simulink subsystem "motor_velocity_loop_model_v2"  (R2023b)
settings: Solver=VariableStepAuto  StartTime=0.0  StopTime=10.0  RelTol=1e-3
values from neighbouring files (symbols this model uses):
  omega_in_bar_dt_max = 628.318530718    [mdl_parameters_int.mat]
  omega_in_bar_dt_min = -1047.1975512    [mdl_parameters_int.mat]
  omega_in_max = 397.935069455    [mdl_parameters_int.mat]
  omega_in_min = 0    [mdl_parameters_int.mat]
  tau_s = 0.0005    [mdl_parameters_int.mat]
undefined symbols (not defined in the file or in its folder): T_omega_in
libraries: cstblocks x2
settings Model: Creator=Previ  LastModifiedBy=Previ

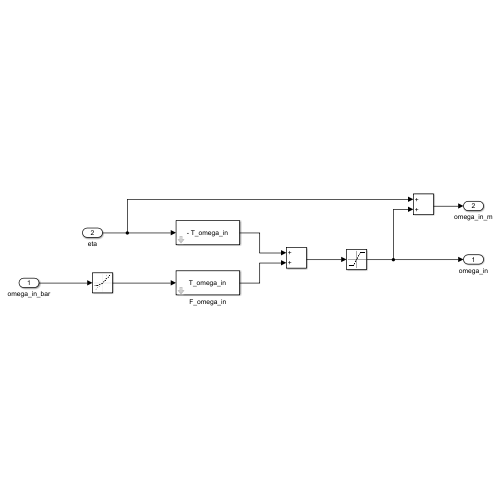
[thumbnail: Simulink's stored preview of the top-level diagram]
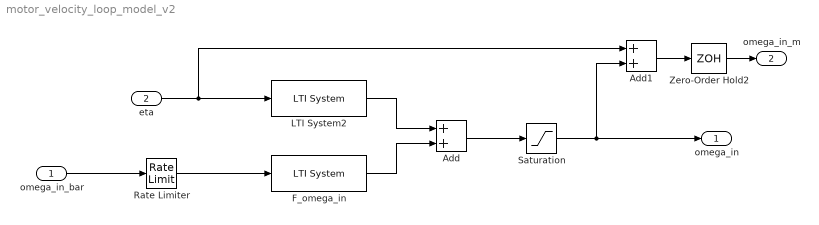
== system motor_velocity_loop_model_v2 ==
  omega_in_bar : Inport  PortDimensions=[1, 1]
  eta : Inport  Port=2  PortDimensions=[1, 1]
  Add : Sum
  Add1 : Sum
  F_omega_in : cstblocks/LTI System  sys=T_omega_in  IC=[]  PadeOrder=0
  LTI System2 : cstblocks/LTI System  sys=- T_omega_in  IC=[]  PadeOrder=0
  Rate Limiter : RateLimiter  RisingSlewLimit=omega_in_bar_dt_max  FallingSlewLimit=omega_in_bar_dt_min  SampleTimeMode=inherited
  Saturation : Saturate  UpperLimit=omega_in_max  LowerLimit=omega_in_min
  Zero-Order Hold2 : ZeroOrderHold  SampleTime=tau_s
  omega_in : Outport  PortDimensions=[1, 1]
  omega_in_m : Outport  Port=2  PortDimensions=[1, 1]
  wires:
  Saturation/1 -> Add1/2, omega_in/1
  Rate Limiter/1 -> F_omega_in/1
  omega_in_bar/1 -> Rate Limiter/1
  Add/1 -> Saturation/1
  eta/1 -> Add1/1, LTI System2/1
  F_omega_in/1 -> Add/2
  LTI System2/1 -> Add/1
  Add1/1 -> Zero-Order Hold2/1
  Zero-Order Hold2/1 -> omega_in_m/1
